simulink model "Simu_Model_vs_Logs"  (R2018b)
settings: Solver=FixedStepAuto  StartTime=0.0  StopTime=60  FixedStep=.00005  RelTol=1e-3
libraries: dsparch4 x2
settings Model: Creator=Lubin Kerhuel  LastModifiedBy=Lubin Kerhuel

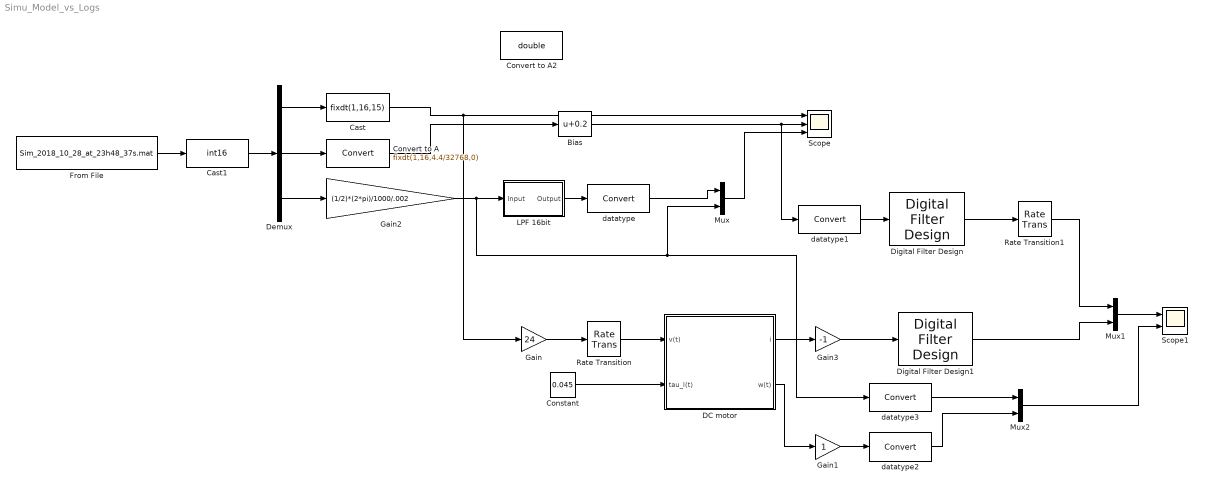
== system Simu_Model_vs_Logs ==
  Bias : Bias  Bias=0.2  SaturateOnIntegerOverflow=on
  Cast : DataTypeConversion  OutDataTypeStr=fixdt(1,16,15)  ConvertRealWorld=Stored Integer (SI)
  Cast1 : DataTypeConversion  OutDataTypeStr=int16
  Constant : Constant  Value=0.045
  Convert to A : DataTypeConversion  OutDataTypeStr=fixdt(1,16,4.4/32768,0)  ConvertRealWorld=Stored Integer (SI)
  Convert to A2 : DataTypeConversion  OutDataTypeStr=double
  DC motor : Subsystem  mask{R=1.22, L=0.0027, Kphi=0.061, J=0.22e-3, F=.0001, C0=0}
      mask prompts: R "Resistance (R) in Ohms"; L "Inductance (L) in H"; Kphi "Back EMF (Kphi) in V/rad/s"; J "J in kgm²"; F "F in N/rad/s"
      mask DialogControl Container3 Prompt: Electrical Parameters
      mask DialogControl Container3_copy Prompt: Mechanical Parameters
  Demux : Demux  Outputs=3
  Digital Filter Design : dsparch4/Digital Filter Design  mwdsp_browser_bugfix_var=off
  Digital Filter Design1 : dsparch4/Digital Filter Design  mwdsp_browser_bugfix_var=off
  From File : FromFile  FileName=Sim_2018_10_28_at_23h48_37s.mat  SampleTime=.00005
  Gain : Gain  Gain=24  OutDataTypeStr=double
  Gain1 : Gain  OutDataTypeStr=double
  Gain2 : Gain  Gain=(1/2)*(2*pi)/1000/.002  OutDataTypeStr=fixdt(1,16,5)  LockScale=on
  Gain3 : Gain  Gain=-1  OutDataTypeStr=double
  "LPF 16bit " : Subsystem  Tag=FilterWizardSubSystem
      settings: ErrorFcn=dspFilterRealizedInBasicElemsAlgLoopErrFcnCallback
  Mux : Mux  Inputs=2
  Mux1 : Mux  Inputs=2
  Mux2 : Mux  Inputs=2
  Rate Transition : RateTransition  Deterministic=off
  Rate Transition1 : RateTransition  Deterministic=off
  Scope : Scope  NumInputPorts=3
  Scope1 : Scope  NumInputPorts=2
  datatype{,1..3} (4 alike) : DataTypeConversion
  wires:
  From File/1 -> Cast1/1
  Demux/1 -> Cast/1
  Demux/2 -> Convert to A/1
  Demux/3 -> Gain2/1
  Cast/1 -> Gain/1, Scope/1
  Convert to A/1 -> Bias/1
  Gain2/1 -> Mux/2, datatype3/1, "LPF 16bit "/1(Input)
  Cast1/1 -> Demux/1
  "LPF 16bit "/1(Output) -> datatype/1
  Mux/1 -> Scope/3
  datatype/1 -> Mux/1
  Gain/1 -> Rate Transition/1
  Constant/1 -> DC motor/2(tau_l(t))
  Rate Transition/1 -> DC motor/1(v(t))
  datatype1/1 -> Digital Filter Design/1
  Rate Transition1/1 -> Mux1/1
  Mux1/1 -> Scope1/1
  DC motor/1(i) -> Gain3/1
  Digital Filter Design/1 -> Rate Transition1/1
  Bias/1 -> datatype1/1, Scope/2
  Digital Filter Design1/1 -> Mux1/2
  DC motor/2(w(t)) -> Gain1/1
  Mux2/1 -> Scope1/2
  datatype2/1 -> Mux2/2
  datatype3/1 -> Mux2/1
  Gain1/1 -> datatype2/1
  Gain3/1 -> Digital Filter Design1/1

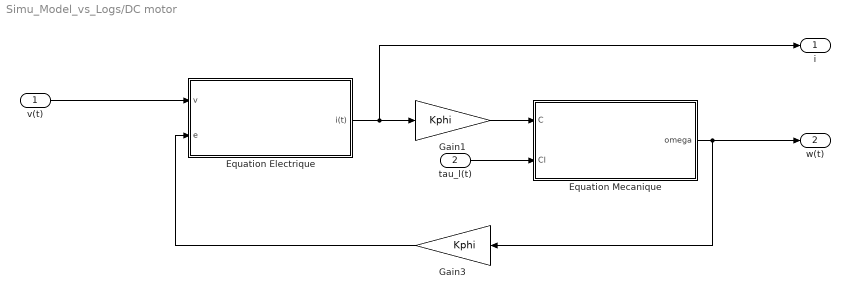
== system Simu_Model_vs_Logs/DC motor ==
  v(t) : Inport
  tau_l(t) : Inport  Port=2
  Equation Electrique : Subsystem
  Equation Mecanique : Subsystem
  Gain1 : Gain  Gain=Kphi
  "Gain3  " : Gain  Gain=Kphi
  i : Outport
  w(t) : Outport  Port=2
  wires:
  "Gain3  "/1 -> Equation Electrique/2(e)
  Gain1/1 -> Equation Mecanique/1(C)
  tau_l(t)/1 -> Equation Mecanique/2(Cl)
  Equation Electrique/1(i(t)) -> i/1, Gain1/1
  Equation Mecanique/1(omega) -> w(t)/1, "Gain3  "/1
  v(t)/1 -> Equation Electrique/1(v)

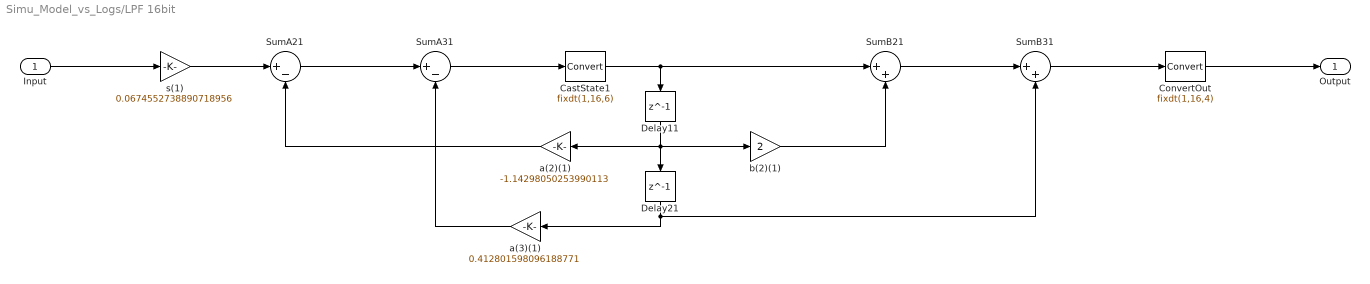
== system Simu_Model_vs_Logs/LPF 16bit  ==
  Input : Inport
  CastState1 : DataTypeConversion  OutDataTypeStr=fixdt(1,16,6)
  ConvertOut : DataTypeConversion  OutDataTypeStr=fixdt(1,16,4)
  Delay11 : Delay  DelayLength=1  InitialCondition=0
  Delay21 : Delay  DelayLength=1  InitialCondition=0
  SumA21 : Sum  Inputs=|+-  AccumDataTypeStr=fixdt(1,16,6)  OutDataTypeStr=fixdt(1,16,6)
  SumA31 : Sum  Inputs=|+-  AccumDataTypeStr=fixdt(1,16,6)  OutDataTypeStr=fixdt(1,16,6)
  SumB21 : Sum  Inputs=|++  AccumDataTypeStr=fixdt(1,16,5)  OutDataTypeStr=fixdt(1,16,5)
  SumB31 : Sum  Inputs=|++  AccumDataTypeStr=fixdt(1,16,4)  OutDataTypeStr=fixdt(1,16,4)
  a(2)(1) : Gain  Gain=-1.14298050253990113  ParamDataTypeStr=fixdt(1,16,14)  OutDataTypeStr=fixdt(1,16,6)
  a(3)(1) : Gain  Gain=0.412801598096188771  ParamDataTypeStr=fixdt(0,16,17)  OutDataTypeStr=fixdt(1,16,8)
  b(2)(1) : Gain  Gain=2  ParamDataTypeStr=fixdt(0,16,14)  OutDataTypeStr=fixdt(1,16,5)
  s(1) : Gain  Gain=0.0674552738890718956  ParamDataTypeStr=fixdt(0,16,19)  OutDataTypeStr=fixdt(1,16,8)
  Output : Outport
  wires:
  s(1)/1 -> SumA21/1
  SumA21/1 -> SumA31/1
  SumA31/1 -> CastState1/1
  CastState1/1 -> SumB21/1, Delay11/1
  SumB21/1 -> SumB31/1
  SumB31/1 -> ConvertOut/1
  a(2)(1)/1 -> SumA21/2
  Delay11/1 -> a(2)(1)/1, b(2)(1)/1, Delay21/1
  b(2)(1)/1 -> SumB21/2
  a(3)(1)/1 -> SumA31/2
  Delay21/1 -> a(3)(1)/1, SumB31/2
  ConvertOut/1 -> Output/1
  Input/1 -> s(1)/1

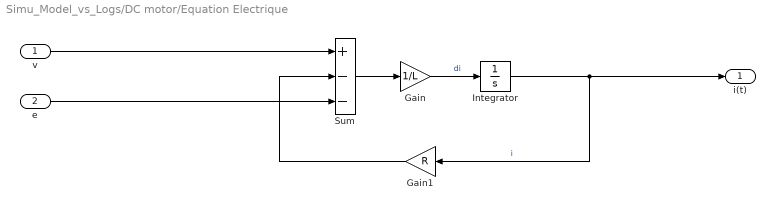
== system Simu_Model_vs_Logs/DC motor/Equation Electrique ==
  v : Inport
  e : Inport  Port=2
  Gain : Gain  Gain=1/L
  Gain1 : Gain  Gain=R
  Integrator : Integrator
  Sum : Sum  Inputs=+--
  i(t) : Outport
  wires:
  Gain1/1 -> Sum/2
  Sum/1 -> Gain/1
  Integrator/1 -> i(t)/1, Gain1/1  "i"
  Gain/1 -> Integrator/1  "di"
  v/1 -> Sum/1
  e/1 -> Sum/3

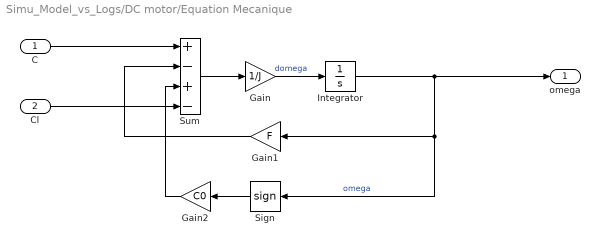
== system Simu_Model_vs_Logs/DC motor/Equation Mecanique ==
  C : Inport
  Cl : Inport  Port=2
  Gain : Gain  Gain=1/J
  Gain1 : Gain  Gain=F
  Gain2 : Gain  Gain=C0
  Integrator : Integrator
  Sign : Signum
  Sum : Sum  Inputs=+-+-
  omega : Outport
  wires:
  Gain/1 -> Integrator/1  "domega"
  Integrator/1 -> Sign/1, Gain1/1, omega/1  "omega"
  Sum/1 -> Gain/1
  Gain1/1 -> Sum/2
  Sign/1 -> Gain2/1
  Gain2/1 -> Sum/3
  C/1 -> Sum/1
  Cl/1 -> Sum/4
